simulink model "sim_example_2_2"  (R2020b)
settings: Solver=ode45  StartTime=0.0  StopTime=100  RelTol=1e-3  EnableMultiTasking=on
settings Model: Creator=Ahmadieh  LastModifiedBy=mojta
settings DataIOCC: LimitDataPoints=on  SaveFormat=Array  ReturnWorkspaceOutputs=off
settings OptimizationCC: LifeSpan=inf
settings DebuggingCC: UnderspecifiedInitializationDetection=Classic  MergeDetectMultiDrivingBlocksExec=none  SolverPrmCheckMsg=warning  SFUnexpectedBacktrackingDiag=warning  SFNoUnconditionalDefaultTransitionDiag=warning  SFExecutionAtInitializationDiag=none  ArithmeticOperatorsInVariantConditions=warning
settings HardwareCC: ProdBitPerPointer=32  ProdBitPerSizeT=32  ProdBitPerPtrDiffT=32  ProdLargestAtomicFloat=None  ProdIntDivRoundTo=Undefined  ProdEndianess=Unspecified  ProdWordSize=32  ProdHWDeviceType=32-bit Generic
settings ModelReferenceCC: PropagateSignalLabelsOutOfModel=off
settings SFSimCC: SimUseLocalCustomCode=off  CustomCodeUndefinedFunction=UseInterfaceOnly
settings RTWCC: RTWUseLocalCustomCode=off
settings CodeAppCC: StateflowObjectComments=on
settings GRTTargetCC: TargetLangStandard=C89/C90 (ANSI)
settings ConfigComp: CovMetricSettings=dw  CovSaveCumulativeToWorkspaceVar=on  CovSaveSingleToWorkspaceVar=on  CovExternalEMLEnable=off

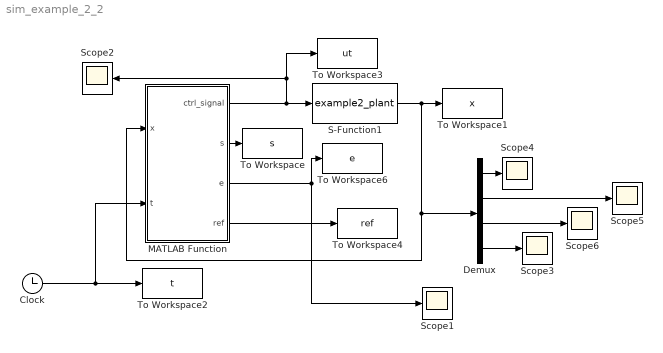
== system sim_example_2_2 ==
  Clock : Clock
  Demux : Demux
  MATLAB Function : MATLAB Function  TreatAsAtomicUnit=on
  S-Function1 : S-Function  FunctionName=example2_plant  SFunctionDeploymentMode=off  EnableBusSupport=off
  Scope{1..6} (6 alike) : Scope
  To Workspace : ToWorkspace  VariableName=s  SampleTime=-1
  To Workspace1 : ToWorkspace  VariableName=x  SampleTime=-1
  To Workspace2 : ToWorkspace  VariableName=t  SampleTime=-1
  To Workspace3 : ToWorkspace  VariableName=ut  SampleTime=-1
  To Workspace4 : ToWorkspace  VariableName=ref  SampleTime=-1
  To Workspace6 : ToWorkspace  VariableName=e  SampleTime=-1
  wires:
  Clock/1 -> MATLAB Function/2(t), To Workspace2/1
  MATLAB Function/1(ctrl_signal) -> S-Function1/1, To Workspace3/1, Scope2/1
  MATLAB Function/2(s) -> To Workspace/1
  S-Function1/1 -> Demux/1, MATLAB Function/1(x), To Workspace1/1
  MATLAB Function/3(e) -> Scope1/1, To Workspace6/1
  MATLAB Function/4(ref) -> To Workspace4/1
  Demux/4 -> Scope3/1
  Demux/1 -> Scope4/1
  Demux/2 -> Scope5/1
  Demux/3 -> Scope6/1

== matlab function sim_example_2_2/MATLAB Function ==
  data: x input; t input; ctrl_signal output; s output; e output; ref output
function [ctrl_signal,s,e,ref] = fcn(x,t)
%#codegen
g=9.8;I=1;L=1;M=1;K=1;J=1;
x1=x(1);x2=x(2);x3=x(3);x4=x(4);
ref=sin(t);dref=cos(t);d2ref=-sin(t);d3ref=-cos(t);d4ref=sin(t);
z1=x1;z2=x2;z3=-M*g*L/I*sin(x1)-K/I*(x1-x3);
z4=-M*g*L/I*x2*cos(x1)-K/I*(x2-x4);
K3=11;K2=38;K1=40;KK=2;eps=0;
s=z4-d3ref+K3*(z3-d2ref)+K2*(z2-dref)+K1*(x1-ref);
ctrl_signal=I*J/K*((M*g*L/I*cos(z1)+K/I+K/J)*z3-...
    M*g*L/I*(z2^2-K/J)*sin(z1)-K3*(z4-d3ref)-K2*(z3-d2ref)...
    -K1*(z2-dref)-KK*sat(s,eps)+d4ref);
e=x1-ref;
end

function y=sat(s,eps)
if abs(s)<eps
    y=s/eps;
else
    y=sign(s);
end
end
